simulink model "lab_modulation_fm_sync_det"  (R2025a)
settings: Solver=VariableStepAuto  StartTime=0.0  StopTime=1  RelTol=1e-3
libraries: dspfdesign x2, dspmathops x1, commanapbnd3 x1
settings Model: Creator=Ksenia Kochneva  LastModifiedBy=Ksenia Kochneva

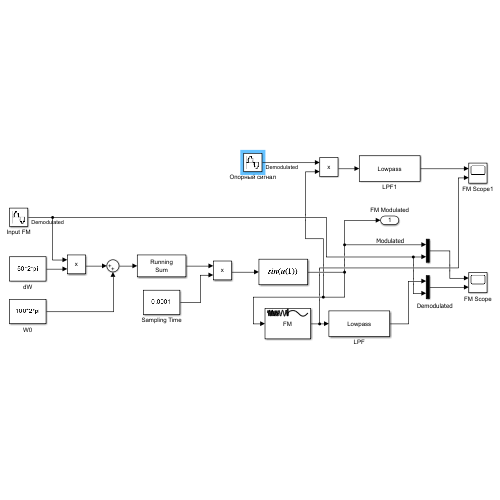
[thumbnail: Simulink's stored preview of the top-level diagram]
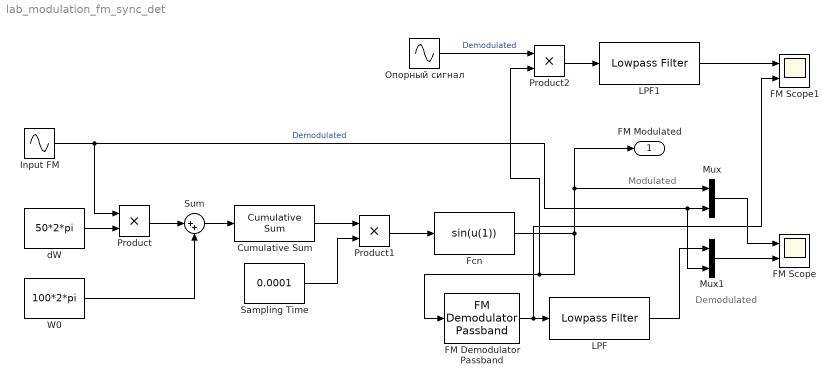
== system lab_modulation_fm_sync_det ==
  note: Demodulated
  note: Modulated
  Cumulative Sum : dspmathops/Cumulative Sum  dim=Channels (running sum)  reset_popup=None  roundingMode=Floor  overflowMode=off  outputDataTypeStr=Inherit: Same as accumulator  outputMin=[]  outputMax=[]  outputLastDataTypeStr=Inherit: Same as accumulator
  FM Demodulator Passband : commanapbnd3/FM Demodulator Passband  Fc=100  Ph=0  Kc=25  Ho=100
  FM Scope : Scope  NumInputPorts=2
      settings: ActiveDisplayYMinimum=-1.2499999999998153  ActiveDisplayYMaximum=1.2499999999999212
  FM Scope1 : Scope  NumInputPorts=2
      settings: ActiveDisplayYMinimum=-3.8397364152037881  ActiveDisplayYMaximum=3.1808721386889021
  Fcn : Fcn  Expr=sin(u(1))
  Input FM : Sin  Frequency=2*2*pi  SampleTime=0.0001
  LPF : dspfdesign/Lowpass Filter  FilterType=FIR  DesignForMinimumOrder=on  FilterOrder=50  PassbandFrequency=0.1  StopbandFrequency=100  PassbandRipple=0.1  StopbandAttenuation=80  SampleRate=44100  SimulateUsing=Interpreted execution  roundingMode=Floor  coeffsDataTypeStr=fixdt(1,16)
  LPF1 : dspfdesign/Lowpass Filter  FilterType=FIR  DesignForMinimumOrder=on  FilterOrder=50  PassbandFrequency=0.1  StopbandFrequency=100  PassbandRipple=0.1  StopbandAttenuation=80  SampleRate=44100  SimulateUsing=Interpreted execution  roundingMode=Floor  coeffsDataTypeStr=fixdt(1,16)
  Mux : Mux  Inputs=2
  Mux1 : Mux  Inputs=2
  Product : Product
  Product1 : Product
  Product2 : Product
  Sampling Time : Constant  Value=0.0001
  Sum : Sum  Inputs=|++
  W0 : Constant  Value=100*2*pi
  dW : Constant  Value=50*2*pi
  Опорный сигнал : Sin  Frequency=95  SampleTime=0.0001
  FM Modulated : Outport
  wires:
  dW/1 -> Product/2
  Fcn/1 -> Product2/2, FM Demodulator Passband/1, FM Modulated/1, Mux/1
  Product1/1 -> Fcn/1
  Mux/1 -> FM Scope/1
  Product/1 -> Sum/1
  W0/1 -> Sum/2
  Mux1/1 -> FM Scope/2
  Input FM/1 -> Product/1, Mux1/2, Mux/2  "Demodulated"
  Cumulative Sum/1 -> Product1/1
  LPF/1 -> Mux1/1
  Sampling Time/1 -> Product1/2
  FM Demodulator Passband/1 -> FM Scope1/2, LPF/1
  Sum/1 -> Cumulative Sum/1
  Product2/1 -> LPF1/1
  LPF1/1 -> FM Scope1/1
  Опорный сигнал/1 -> Product2/1  "Demodulated"
